simulink model "MultiSatellite_GNC_sire"  (R2021a)
settings: Solver=VariableStepAuto  StartTime=0.0  StopTime=150  RelTol=1e-3
libraries: simulink x4
settings Model: Creator=akshy  LastModifiedBy=akshy

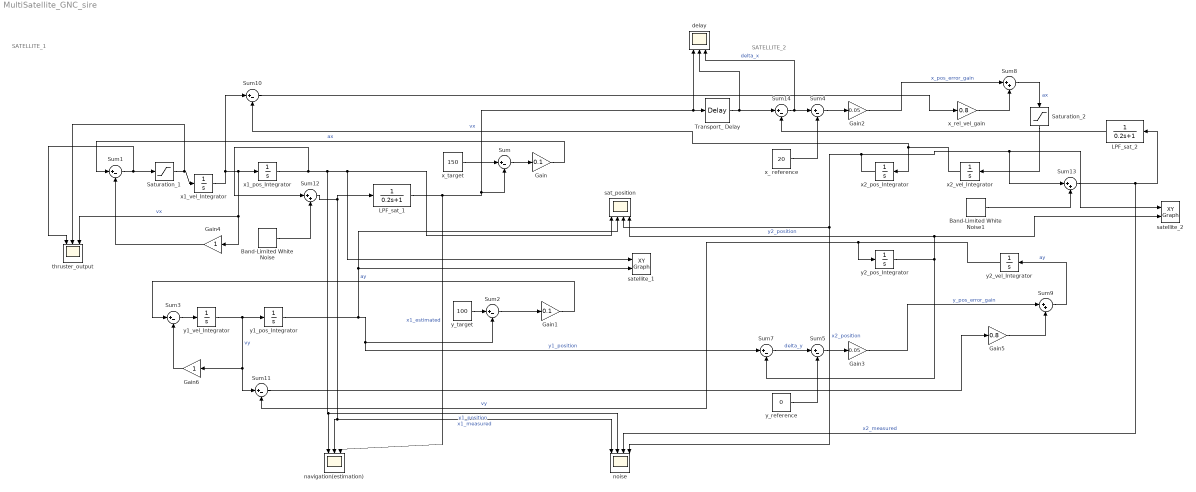
== system MultiSatellite_GNC_sire ==
  note: SATELLITE_1
  note: SATELLITE_2
  " LPF_sat_1" : TransferFcn  Denominator=[0.2 1]
  " LPF_sat_2" : TransferFcn  Denominator=[0.2 1]
  Band-Limited White Noise : simulink/Sources/Band-Limited White Noise  Cov=[5]  Ts=0.1  seed=[23341]
  Band-Limited White Noise1 : simulink/Sources/Band-Limited White Noise  Cov=[10]  Ts=0.1  seed=[23341]
  Gain : Gain  Gain=0.1
  Gain1 : Gain  Gain=0.1
  Gain2 : Gain  Gain=0.05
  Gain3 : Gain  Gain=0.05
  Gain4 : Gain
  Gain5 : Gain  Gain=0.8
  Gain6 : Gain
  Saturation_1 : Saturate  UpperLimit=2  LowerLimit=-2
  Saturation_2 : Saturate  UpperLimit=2  LowerLimit=-2
  Sum{,1..5,7,10..11,14} (10 alike) : Sum  Inputs=|+-
  Sum{8..9,12..13} (4 alike) : Sum  Inputs=|++
  Transport_ Delay : TransportDelay
  delay : Scope  NumInputPorts=3
  navigation(estimation) : Scope  NumInputPorts=3
  noise : Scope  NumInputPorts=4
  sat_position : Scope  NumInputPorts=4
  satellite_1 : simulink/Sinks/XY Graph  xmin=0  xmax=160  ymin=0  ymax=120  st=-1
  satellite_2 : simulink/Sinks/XY Graph  xmin=0  xmax=160  ymin=0  ymax=120  st=-1
  thruster_output : Scope  NumInputPorts=3
  x1_pos_Integrator : Integrator
  x1_vel_Integrator : Integrator
  x2_pos_Integrator : Integrator  InitialCondition=-20
  x2_vel_Integrator : Integrator
  x_ reference : Constant  Value=20
  x_rel_vel_gain : Gain  Gain=0.8
  x_target : Constant  Value=150
  y1_pos_Integrator : Integrator
  y1_vel_Integrator : Integrator
  y2_pos_Integrator : Integrator
  y2_vel_Integrator : Integrator
  y_reference : Constant  Value=0
  y_target : Constant  Value=100
  wires:
  Gain5/1 -> Sum9/2
  Gain2/1 -> Sum8/1  "x_pos_error_gain"
  y2_vel_Integrator/1 -> Sum11/2, y2_pos_Integrator/1  "vy"
  x2_pos_Integrator/1 -> Sum13/1, satellite_2/1, sat_position/3, noise/4  "x2_position"
  y2_pos_Integrator/1 -> Sum7/2, satellite_2/2, sat_position/4  "y2_position"
  Sum7/1 -> Sum5/1  "delta_y"
  Sum9/1 -> y2_vel_Integrator/1  "ay"
  x_ reference/1 -> Sum4/2
  Sum5/1 -> Gain3/1
  x_rel_vel_gain/1 -> Sum8/2
  y_reference/1 -> Sum5/2
  x2_vel_Integrator/1 -> Sum10/2, x2_pos_Integrator/1  "vx"
  Sum8/1 -> Saturation_2/1  "ax"
  Sum14/1 -> delay/3, Sum4/1  "delta_x"
  Sum4/1 -> Gain2/1
  Gain3/1 -> Sum9/1  "y_pos_error_gain"
  Band-Limited White Noise1/1 -> Sum13/2
  Sum13/1 -> " LPF_sat_2"/1, noise/3  "x2_measured"
  Sum10/1 -> x_rel_vel_gain/1
  Sum11/1 -> Gain5/1
  Gain6/1 -> Sum3/2
  Gain4/1 -> Sum1/2
  y_target/1 -> Sum2/1
  x_target/1 -> Sum/1
  Gain/1 -> Sum1/1  "ax"
  Sum/1 -> Gain/1
  Gain1/1 -> Sum3/1  "ay"
  Band-Limited White Noise/1 -> Sum12/2
  y1_vel_Integrator/1 -> Gain6/1, Sum11/1, y1_pos_Integrator/1  "vy"
  Sum3/1 -> y1_vel_Integrator/1
  Sum12/1 -> " LPF_sat_1"/1, noise/1, navigation(estimation)/2  "x1_measured"
  Sum1/1 -> thruster_output/1, Saturation_1/1
  x1_vel_Integrator/1 -> Sum10/1, thruster_output/3, Gain4/1, x1_pos_Integrator/1  "vx"
  Sum2/1 -> Gain1/1
  x1_pos_Integrator/1 -> sat_position/1, satellite_1/1, noise/2, navigation(estimation)/1, Sum12/1  "x1_position"
  y1_pos_Integrator/1 -> Sum7/1, Sum2/2, sat_position/2, satellite_1/2  "y1_position"
  " LPF_sat_1"/1 -> Sum/2, Transport_ Delay/1, delay/1, navigation(estimation)/3  "x1_estimated"
  " LPF_sat_2"/1 -> Sum14/2
  Saturation_1/1 -> thruster_output/2, x1_vel_Integrator/1
  Saturation_2/1 -> x2_vel_Integrator/1
  Transport_ Delay/1 -> delay/2, Sum14/1
